simulink model "simulink_model"  (R2023a)
settings: Solver=VariableStepAuto  StartTime=0.0  StopTime=100  RelTol=1e-1
InitFcn:
  | m = 0.0489; % Mass of the drone (kg)
  | d = 0.00116; % Torque constant of one motor (N*m / s^2)
  | b = 4*1e-5; % Thrust constant of one motor (N / s^2)
  | Ixx = 48932*1e-9; % Drone inertia around the xx axis (Kg * m^2)
  | Iyy = 49929*1e-9; % Drone inertia around the yy axis (Kg * m^2)
  | Izz = 99299*1e-9; % Drone inertia around the zz axis (Kg * m^2)
  | l = 0.116 / 2; % Lenght from the motor to the mid point (m)
  | Jr = 729*1e-9; % Rotor inertia (Kg * m^2)
  | Ax = 0; % Air resistance from axis X (kg / s)
  | Ay = 0; % Air resistance from axis Y (kg / s)
  | Az = 0; % Air resistance from axis Z (kg / s)
  | g = 9.81; % The accelaration from gravity (m / s^2)
  | 
  | %Theta PID
  | Theta_P = 0;%2 * 0.6;
  | Theta_I = 0;%0.132 / 2;
  | Theta_D = 0;%0.132 / 8;
  | 
  | %Phi PID
  | Phi_P = 0;
  | Phi_I = 0;
  | Phi_D = 0;
  | 
  | %Psi_dot PID
  | Psi_dot_P = 0;
  | Psi_dot_I = 0;
  | Psi_dot_D = 0;
  | 
  | %Without noise
  | %Starting calibration Kp = 0.4
  | Z_P = 0.7 * 0.6; %0.8 * 0.6
  | Z_I = 0.99 / 2;
  | Z_D = 1.3 / 8;
libraries: slpidlib x2, sim3dlib x1, uavsim3dlib x1
settings Model: Creator=Artis  LastModifiedBy=Artis
settings OptimizationCC: ReuseModelBlockBuffer=off

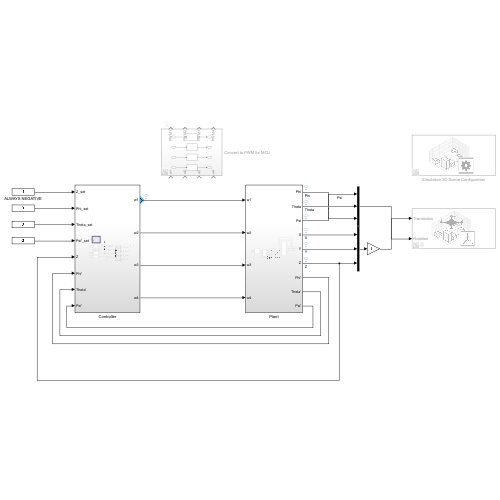
[thumbnail: Simulink's stored preview of the top-level diagram]
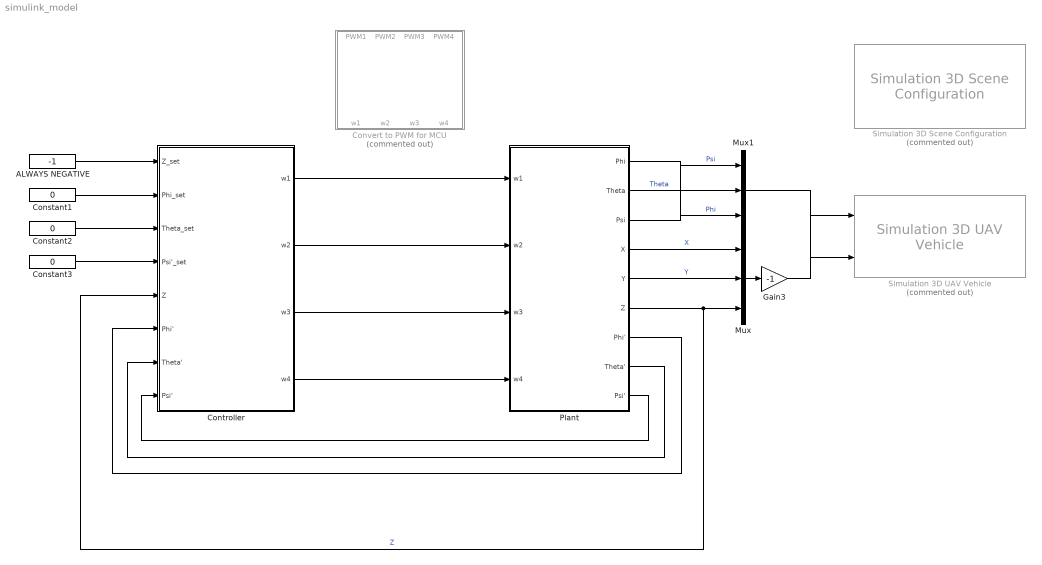
== system simulink_model ==
  ALWAYS NEGATIVE : Constant  Value=-1
  Constant1 : Constant  Value=0
  Constant2 : Constant  Value=0
  Constant3 : Constant  Value=0
  Controller : Subsystem
  Convert to PWM for MCU : Subsystem  Commented=on
  Gain3 : Gain  Gain=-1
  Mux : Mux  Inputs=3
  Mux1 : Mux  Inputs=3
  Plant : Subsystem
  Simulation 3D Scene Configuration : sim3dlib/Simulation 3D Scene Configuration  Priority=0  Commented=on  ProjectFormat=Default Scenes  SceneDesc=US city block  ProjectName=C:\Program Files\MATLAB\R2023a\toolbox\shared\sim3d_projects\automotive_project\UE4\WindowsNoEditor\VehicleSimulation.exe  ScenePath=/Game/Maps/USCityBlock  EnableOpenDRIVE=off  vehTagList={'Scene Origin';'SimulinkVehicle1'}  vehTag=SimulinkVehicle1  OpVisEn=off  Ts=1/60  EnableWindow=on  EnableRemoteAccess=off  EnableWeather=off  SunAltitude=40.0  SunAzimuth=90  clouds=10  wind=1  fog=0  rain=0  EnableGeospatial=off  OriginHeight=200  OriginLatitude=40.744652  OriginLongitude=-73.988864  MapStyle=Aerial  AdditionalAssetIDs=[]  UseAdvancedSunSky=off  SolarTime=11  TimeZone=-5  Day=21  Month=9  Year=2022  UseDaylightSavingTime=on  DSTStartDay=10  DSTStartMonth=3  DSTEndDay=3  DSTEndMonth=11  DSTSwitchHour=2  sensorTag=MainCamera1  sensorId=1  sensorName=MainCamera1  mountLoc=Origin  offsetFlag=off  tmountOffset=[0, 0, 0]  rmountOffset=[0, 0, 0]  HorizontalResolution=1280  VerticalResolution=720  HorizontalFOV=60  mountPoint=[0 0 0]  mountOrientation=[0 0 0]  aMode=4  ID=1  GeoTrigger=Inactive
      settings: LibrarySourceBlock=uavsim3dlib/Simulation 3D Scene Configuration
  Simulation 3D UAV Vehicle : uavsim3dlib/Simulation 3D UAV Vehicle  Priority=-1  Commented=on  Mesh=Quadrotor  MeshPath=/MathWorksUAVContent/UAVs/HexaRotorUAV/HexaRotor.HexaRotor  Color=Black  ActorName=SimulinkVehicle1  UseGlobalFrame=off  InitialTranslation=[0 0 0]  InitialRotation=[0 0 0]  InitialTranslationGlobal=[0 0 0]  InitialGeoOrigin=[0 0 0]  InitialRotationGlobal=[0 0 0]  SampleTime=-1  ActorType=SimulinkVehicle  ID=1  aMode=4  ActorTag=SimulinkVehicle1
  wires:
  Plant/6(Z) -> Controller/5(Z), Mux/3  "Z"
  Plant/5(Y) -> Mux/2  "Y"
  Plant/3(Psi) -> Mux1/1  "Psi"
  Plant/2(Theta) -> Mux1/2  "Theta"
  Plant/1(Phi) -> Mux1/3  "Phi"
  Plant/4(X) -> Mux/1  "X"
  Mux/1 -> Gain3/1
  Mux1/1 -> Simulation 3D UAV Vehicle/2
  Gain3/1 -> Simulation 3D UAV Vehicle/1
  ALWAYS NEGATIVE/1 -> Controller/1(Z_set)
  Constant1/1 -> Controller/2(Phi_set)
  Constant2/1 -> Controller/3(Theta_set)
  Constant3/1 -> Controller/4(Psi'_set)
  Plant/9(Psi') -> Controller/8(Psi')
  Controller/1(w1) -> Plant/1(w1)
  Controller/2(w2) -> Plant/2(w2)
  Controller/4(w4) -> Plant/4(w4)
  Controller/3(w3) -> Plant/3(w3)
  Plant/7(Phi') -> Controller/6(Phi')
  Plant/8(Theta') -> Controller/7(Theta')

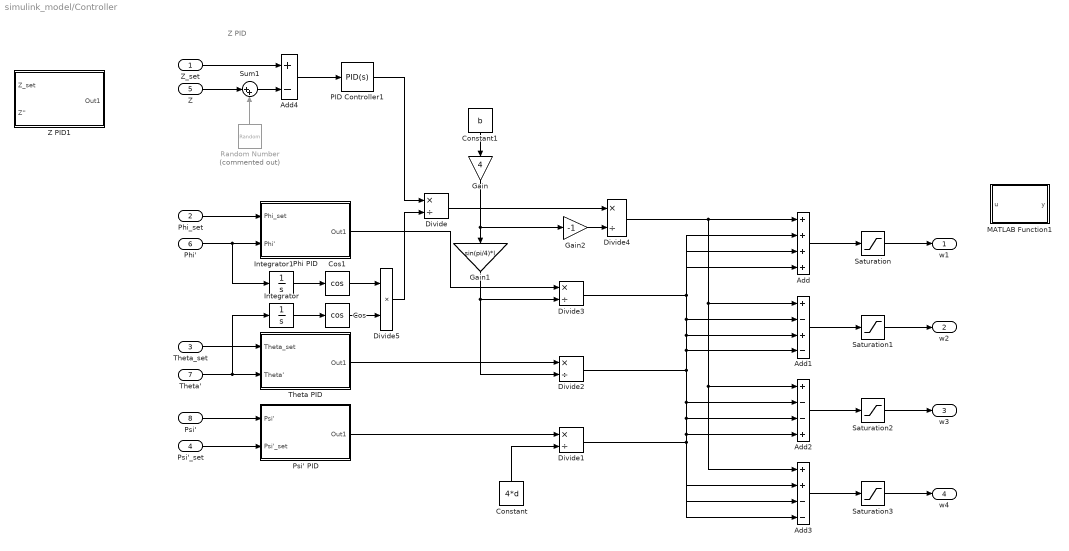
== system simulink_model/Controller ==
  note: Z PID
  Z_set : Inport
  Phi_set : Inport  Port=2
  Theta_set : Inport  Port=3
  Psi'_set : Inport  Port=4
  Z : Inport  Port=5
  Phi' : Inport  Port=6
  Theta' : Inport  Port=7
  Psi' : Inport  Port=8
  Add : Sum  Inputs=++++
  Add1 : Sum  Inputs=+-+-
  Add2 : Sum  Inputs=+--+
  Add3 : Sum  Inputs=++--
  Add4 : Sum  Inputs=+-
  Constant : Constant  Value=4*d
  Constant1 : Constant  Value=b
  Cos : Trigonometry  Operator=cos
  Cos1 : Trigonometry  Operator=cos
  Divide{,1..4} (5 alike) : Product  Inputs=*/
  Divide5 : Product  Inputs=**
  Gain : Gain  Gain=4
  Gain1 : Gain  Gain=sin(pi/4)*l
  Gain2 : Gain  Gain=-1
  Integrator : Integrator
  Integrator1 : Integrator
  MATLAB Function1 : MATLAB Function  TreatAsAtomicUnit=on
  PID Controller1 : slpidlib/PID Controller  Controller=PID  Form=Parallel  TimeDomain=Continuous-time  UseExternalTs=off  SampleTime=-1  IntegratorMethod=Forward Euler  FilterMethod=Forward Euler  ControllerParametersSource=internal  P=0.00907971597395873  I=0.000425064890164197  UseKiTs=off  D=0.0476247360001517  N=5.45397025421619  UseFilter=on  TunerSelectOption=Transfer Function Based (PID Tuner App)  InitialConditionSource=internal  InitialConditionForIntegrator=0  InitialConditionForFilter=0  DifferentiatorICPrevScaledInput=0  ExternalReset=none  TrackingMode=off  Kt=1  LimitOutput=off  SatLimitsSource=internal  UpperSaturationLimit=inf  LowerSaturationLimit=-inf  LinearizeAsGain=on  AntiWindupMode=none  Kb=1  LimitIntegrator=off  UpperIntegratorSaturationLimit=inf  LowerIntegratorSaturationLimit=-inf  POutMin=[]  POutMax=[]  IOutMin=[]  IOutMax=[]  DOutMin=[]  DOutMax=[]  NOutMin=[]  NOutMax=[]  SumOutMin=[]  SumOutMax=[]  SaturationOutMin=[]  SaturationOutMax=[]  PParamMin=[]  PParamMax=[]  IParamMin=[]  IParamMax=[]  DParamMin=[]  DParamMax=[]  NParamMin=[]  NParamMax=[]  KbParamMin=[]  KbParamMax=[]  KtParamMin=[]  KtParamMax=[]  KbOutMin=[]  KbOutMax=[]  KtOutMin=[]  KtOutMax=[]  IntegratorOutMin=[]  IntegratorOutMax=[]  FilterOutMin=[]  FilterOutMax=[]  SumI1OutMin=[]  SumI1OutMax=[]  SumI2OutMin=[]  SumI2OutMax=[]  SumI3OutMin=[]  SumI3OutMax=[]  SumI4OutMin=[]  SumI4OutMax=[]  SumDOutMin=[]  SumDOutMax=[]  DifferentiatorOutMin=[]  DifferentiatorOutMax=[]  FilterDiffOutCoefMin=[]  FilterDiffOutCoefMax=[]  ReciprocalOutMin=[]  ReciprocalOutMax=[]  SumDenOutMin=[]  SumDenOutMax=[]  SumNumOutMin=[]  SumNumOutMax=[]  DivideOutMin=[]  DivideOutMax=[]  UdiffTsProdOutMin=[]  UdiffTsProdOutMax=[]  NTsProdOutMin=[]  NTsProdOutMax=[]  UintegralTsProdOutMin=[]  UintegralTsProdOutMax=[]  UngainTsProdOutMin=[]  UngainTsProdOutMax=[]  ClampingZeroOutDataTypeStr=Inherit: Inherit via back propagation  ClampingZeroOutMin=[]  ClampingZeroOutMax=[]  FilterDenConstantOutDataTypeStr=Inherit: Inherit via back propagation  FilterDenConstantOutMin=[]  FilterDenConstantOutMax=[]  PCopyOutDataTypeStr=Inherit: Inherit via back propagation  PCopyOutMin=[]  PCopyOutMax=[]  NCopyOutDataTypeStr=Inherit: Inherit via back propagation  NCopyOutMin=[]  NCopyOutMax=[]  IntegratorContinuousStateAttributes=''  IntegratorStateMustResolveToSignalObject=off  IntegratorRTWStateStorageClass=Auto  FilterContinuousStateAttributes=''  FilterStateMustResolveToSignalObject=off  FilterRTWStateStorageClass=Auto  ParallelPVariant=InternalParameters  IdealPVariant=Disabled  IVariant=InternalParameters  DVariant=InternalParameters  IntegratorVariant=Continuous  SatVariant=Disabled  AWVariant=Passthrough  PCopyVariant=Disabled  TRVariant=Disabled  FdbkBlocksVariant=Forward  IdealPFdbkVariant=Disabled  SatFdbkVariant=Disabled  DerivativeFilterVariant=ContFilter  NVariant=InternalParameters  NCopyVariant=Disabled  FilterICVariant=InternalICsFilter  IntegratorICVariant=InternalICs  ExternalResetVariant=Disabled  TRSumVariant=Passthrough  SumFdbkVariant=Disabled  SumVariant=Sum_PID  TsampFilterVariant=InternalTs  TsampNgainVariant=Passthrough  TsampIntegralVariant=Passthrough  ExternalSaturationOutDataTypeStr=Inherit: Same as second input
  Phi PID : Subsystem
  Psi' PID : Subsystem
  Random Number : RandomNumber  Commented=on  Variance=0.001  SampleTime=0.01
  Saturation{,1..3} (4 alike) : Saturate  UpperLimit=3500  LowerLimit=0
  Sum1 : Sum  Inputs=|++
  Theta PID : Subsystem
  Z PID1 : Subsystem
  w1 : Outport
  w2 : Outport  Port=2
  w3 : Outport  Port=3
  w4 : Outport  Port=4
  wires:
  Psi'/1 -> Psi' PID/1(Psi')
  Psi'_set/1 -> Psi' PID/2(Psi'_set)
  Phi_set/1 -> Phi PID/1(Phi_set)
  Phi'/1 -> Integrator1/1, Phi PID/2(Phi')
  Theta'/1 -> Integrator/1, Theta PID/2(Theta')
  Theta_set/1 -> Theta PID/1(Theta_set)
  PID Controller1/1 -> Divide/1
  Integrator/1 -> Cos/1
  Integrator1/1 -> Cos1/1
  Divide5/1 -> Divide/2
  Cos1/1 -> Divide5/1
  Cos/1 -> Divide5/2
  Constant1/1 -> Gain/1
  Gain/1 -> Gain1/1, Gain2/1
  Gain2/1 -> Divide4/2
  Gain1/1 -> Divide3/2, Divide2/2
  Constant/1 -> Divide1/2
  Psi' PID/1(Out1) -> Divide1/1
  Divide1/1 -> Add/4, Add1/4, Add2/4, Add3/4
  Divide3/1 -> Add2/2, Add3/2, Add1/2, Add/2
  Divide2/1 -> Add2/3, Add3/3, Add/3, Add1/3
  Divide4/1 -> Add2/1, Add3/1, Add1/1, Add/1
  Theta PID/1(Out1) -> Divide2/1
  Phi PID/1(Out1) -> Divide3/1
  Divide/1 -> Divide4/1
  Add/1 -> Saturation/1
  Add1/1 -> Saturation1/1
  Add2/1 -> Saturation2/1
  Add3/1 -> Saturation3/1
  Saturation/1 -> w1/1
  Saturation1/1 -> w2/1
  Saturation2/1 -> w3/1
  Saturation3/1 -> w4/1
  Sum1/1 -> Add4/2
  Z/1 -> Sum1/1
  Random Number/1 -> Sum1/2
  Add4/1 -> PID Controller1/1
  Z_set/1 -> Add4/1

== system simulink_model/Convert to PWM for MCU ==
  w1 : Inport
  w2 : Inport  Port=2
  w3 : Inport  Port=3
  w4 : Inport  Port=4
  MATLAB Function : MATLAB Function  TreatAsAtomicUnit=on
  MATLAB Function1 : MATLAB Function  TreatAsAtomicUnit=on
  MATLAB Function2 : MATLAB Function  TreatAsAtomicUnit=on
  MATLAB Function3 : MATLAB Function  TreatAsAtomicUnit=on
  PWM1 : Outport
  PWM2 : Outport  Port=2
  PWM3 : Outport  Port=3
  PWM4 : Outport  Port=4
  wires:
  MATLAB Function1/1(y) -> PWM2/1
  w1/1 -> MATLAB Function/1(x)
  w3/1 -> MATLAB Function2/1(x)
  w2/1 -> MATLAB Function1/1(x)
  MATLAB Function2/1(y) -> PWM3/1
  MATLAB Function/1(y) -> PWM1/1
  MATLAB Function3/1(y) -> PWM4/1
  w4/1 -> MATLAB Function3/1(x)

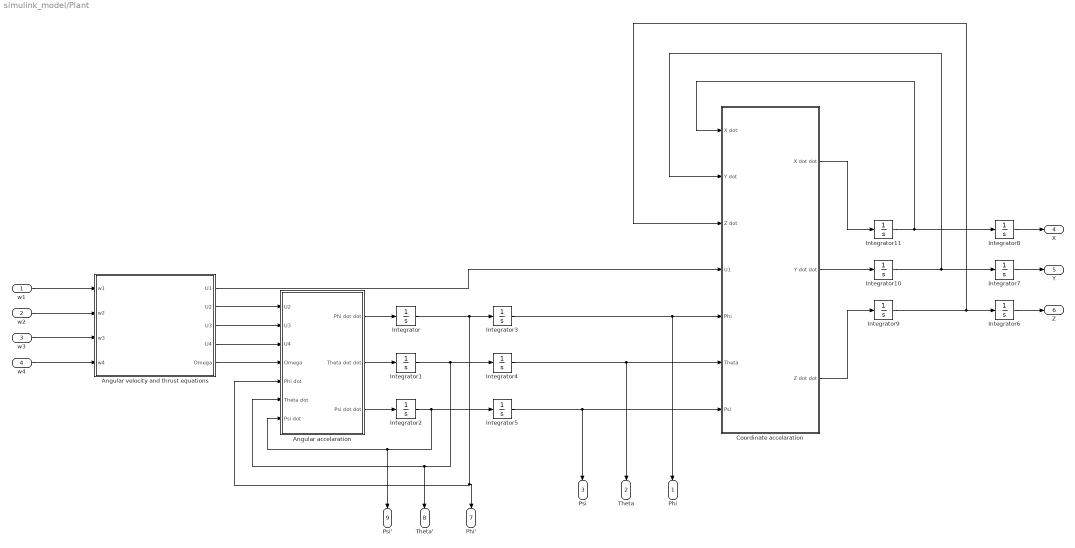
== system simulink_model/Plant ==
  w1 : Inport
  w2 : Inport  Port=2
  w3 : Inport  Port=3
  w4 : Inport  Port=4
  Angular accelaration : Subsystem
  Angular velocity and thrust equations : Subsystem
  Coordinate accelaration : Subsystem
  Integrator{,1..5,7..11} (11 alike) : Integrator
  Integrator6 : Integrator  LimitOutput=on  UpperSaturationLimit=0
  Phi : Outport
  Theta : Outport  Port=2
  Psi : Outport  Port=3
  X : Outport  Port=4
  Y : Outport  Port=5
  Z : Outport  Port=6
  Phi' : Outport  Port=7
  Theta' : Outport  Port=8
  Psi' : Outport  Port=9
  wires:
  w1/1 -> Angular velocity and thrust equations/1(w1)
  w3/1 -> Angular velocity and thrust equations/3(w3)
  Angular velocity and thrust equations/5(Omega) -> Angular accelaration/4(Omega)
  Angular velocity and thrust equations/4(U4) -> Angular accelaration/3(U4)
  Angular velocity and thrust equations/3(U3) -> Angular accelaration/2(U3)
  Angular velocity and thrust equations/2(U2) -> Angular accelaration/1(U2)
  Angular accelaration/1(Phi dot dot) -> Integrator/1
  Angular accelaration/2(Theta dot dot) -> Integrator1/1
  Angular accelaration/3(Psi dot dot) -> Integrator2/1
  Integrator/1 -> Integrator3/1, Phi'/1, Angular accelaration/5(Phi dot)
  Integrator1/1 -> Integrator4/1, Theta'/1, Angular accelaration/6(Theta dot)
  Integrator2/1 -> Integrator5/1, Psi'/1, Angular accelaration/7(Psi dot)
  Integrator4/1 -> Coordinate accelaration/6(Theta), Theta/1
  Integrator3/1 -> Coordinate accelaration/5(Phi), Phi/1
  Integrator5/1 -> Coordinate accelaration/7(Psi), Psi/1
  Angular velocity and thrust equations/1(U1) -> Coordinate accelaration/4(U1)
  Integrator6/1 -> Z/1
  Integrator7/1 -> Y/1
  Integrator8/1 -> X/1
  Integrator10/1 -> Integrator7/1, Coordinate accelaration/2(Y dot)
  Integrator9/1 -> Integrator6/1, Coordinate accelaration/3(Z dot)
  Integrator11/1 -> Integrator8/1, Coordinate accelaration/1(X dot)
  Coordinate accelaration/1(X dot dot) -> Integrator11/1
  Coordinate accelaration/2(Y dot dot) -> Integrator10/1
  Coordinate accelaration/3(Z dot dot) -> Integrator9/1
  w2/1 -> Angular velocity and thrust equations/2(w2)
  w4/1 -> Angular velocity and thrust equations/4(w4)

== system simulink_model/Controller/Phi PID ==
  Phi_set : Inport
  Phi' : Inport  Port=2
  Add : Sum  Inputs=+-
  Add1 : Sum  Inputs=++-
  Gain : Gain  Gain=Phi_P
  Gain1 : Gain  Gain=Phi_I
  Gain2 : Gain  Gain=Phi_D
  Integrator : Integrator
  Integrator1 : Integrator
  Out1 : Outport
  wires:
  Phi_set/1 -> Add/1
  Add1/1 -> Out1/1
  Gain/1 -> Add1/1
  Add/1 -> Gain/1, Integrator/1
  Integrator/1 -> Gain1/1
  Gain1/1 -> Add1/2
  Gain2/1 -> Add1/3
  Phi'/1 -> Gain2/1, Integrator1/1
  Integrator1/1 -> Add/2

== system simulink_model/Controller/Psi' PID ==
  Psi' : Inport
  Psi'_set : Inport  Port=2
  Add : Sum  Inputs=-+
  Add1 : Sum  Inputs=+++
  Derivative : Derivative
  Gain : Gain  Gain=Psi_dot_P
  Gain1 : Gain  Gain=Psi_dot_I
  Gain2 : Gain  Gain=Psi_dot_D
  Integrator : Integrator
  Out1 : Outport
  wires:
  Psi'/1 -> Add/1
  Psi'_set/1 -> Add/2
  Add1/1 -> Out1/1
  Gain/1 -> Add1/1
  Integrator/1 -> Gain1/1
  Gain1/1 -> Add1/2
  Gain2/1 -> Add1/3
  Add/1 -> Derivative/1, Gain/1, Integrator/1
  Derivative/1 -> Gain2/1

== system simulink_model/Controller/Theta PID ==
  Theta_set : Inport
  Theta' : Inport  Port=2
  Add : Sum  Inputs=+-
  Add1 : Sum  Inputs=++-
  Gain : Gain  Gain=Theta_P
  Gain1 : Gain  Gain=Theta_I
  Gain2 : Gain  Gain=Theta_D
  Integrator : Integrator
  Integrator1 : Integrator
  Random Number : RandomNumber  SampleTime=0.1
  Sum : Sum  Inputs=|++
  Out1 : Outport
  wires:
  Theta_set/1 -> Add/1
  Add1/1 -> Out1/1
  Gain/1 -> Add1/1
  Add/1 -> Sum/1, Integrator/1
  Integrator/1 -> Gain1/1
  Gain1/1 -> Add1/2
  Gain2/1 -> Add1/3
  Theta'/1 -> Gain2/1, Integrator1/1
  Integrator1/1 -> Add/2
  Sum/1 -> Gain/1
  Random Number/1 -> Sum/2

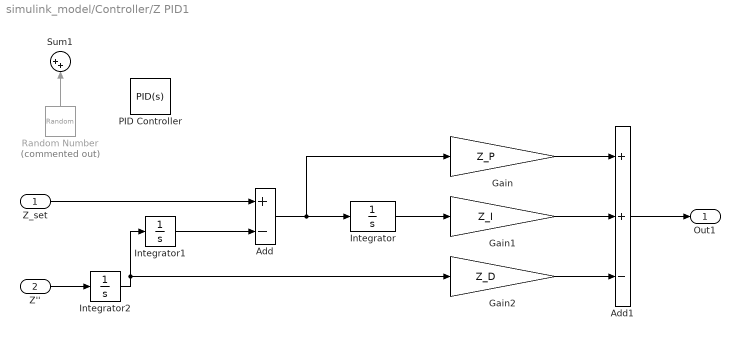
== system simulink_model/Controller/Z PID1 ==
  Z_set : Inport
  Z'' : Inport  Port=2
  Add : Sum  Inputs=+-
  Add1 : Sum  Inputs=++-
  Gain : Gain  Gain=Z_P
  Gain1 : Gain  Gain=Z_I
  Gain2 : Gain  Gain=Z_D
  Integrator : Integrator
  Integrator1 : Integrator  LimitOutput=on  UpperSaturationLimit=0
  Integrator2 : Integrator
  PID Controller : slpidlib/PID Controller  Controller=PID  Form=Parallel  TimeDomain=Continuous-time  UseExternalTs=off  SampleTime=-1  IntegratorMethod=Forward Euler  FilterMethod=Forward Euler  ControllerParametersSource=internal  P=1  I=1  UseKiTs=off  D=0  N=100  UseFilter=on  TunerSelectOption=Transfer Function Based (PID Tuner App)  InitialConditionSource=internal  InitialConditionForIntegrator=0  InitialConditionForFilter=0  DifferentiatorICPrevScaledInput=0  ExternalReset=none  TrackingMode=off  Kt=1  LimitOutput=off  SatLimitsSource=internal  UpperSaturationLimit=inf  LowerSaturationLimit=-inf  LinearizeAsGain=on  AntiWindupMode=none  Kb=1  LimitIntegrator=off  UpperIntegratorSaturationLimit=inf  LowerIntegratorSaturationLimit=-inf  POutMin=[]  POutMax=[]  IOutMin=[]  IOutMax=[]  DOutMin=[]  DOutMax=[]  NOutMin=[]  NOutMax=[]  SumOutMin=[]  SumOutMax=[]  SaturationOutMin=[]  SaturationOutMax=[]  PParamMin=[]  PParamMax=[]  IParamMin=[]  IParamMax=[]  DParamMin=[]  DParamMax=[]  NParamMin=[]  NParamMax=[]  KbParamMin=[]  KbParamMax=[]  KtParamMin=[]  KtParamMax=[]  KbOutMin=[]  KbOutMax=[]  KtOutMin=[]  KtOutMax=[]  IntegratorOutMin=[]  IntegratorOutMax=[]  FilterOutMin=[]  FilterOutMax=[]  SumI1OutMin=[]  SumI1OutMax=[]  SumI2OutMin=[]  SumI2OutMax=[]  SumI3OutMin=[]  SumI3OutMax=[]  SumI4OutMin=[]  SumI4OutMax=[]  SumDOutMin=[]  SumDOutMax=[]  DifferentiatorOutMin=[]  DifferentiatorOutMax=[]  FilterDiffOutCoefMin=[]  FilterDiffOutCoefMax=[]  ReciprocalOutMin=[]  ReciprocalOutMax=[]  SumDenOutMin=[]  SumDenOutMax=[]  SumNumOutMin=[]  SumNumOutMax=[]  DivideOutMin=[]  DivideOutMax=[]  UdiffTsProdOutMin=[]  UdiffTsProdOutMax=[]  NTsProdOutMin=[]  NTsProdOutMax=[]  UintegralTsProdOutMin=[]  UintegralTsProdOutMax=[]  UngainTsProdOutMin=[]  UngainTsProdOutMax=[]  ClampingZeroOutDataTypeStr=Inherit: Inherit via back propagation  ClampingZeroOutMin=[]  ClampingZeroOutMax=[]  FilterDenConstantOutDataTypeStr=Inherit: Inherit via back propagation  FilterDenConstantOutMin=[]  FilterDenConstantOutMax=[]  PCopyOutDataTypeStr=Inherit: Inherit via back propagation  PCopyOutMin=[]  PCopyOutMax=[]  NCopyOutDataTypeStr=Inherit: Inherit via back propagation  NCopyOutMin=[]  NCopyOutMax=[]  IntegratorContinuousStateAttributes=''  IntegratorStateMustResolveToSignalObject=off  IntegratorRTWStateStorageClass=Auto  FilterContinuousStateAttributes=''  FilterStateMustResolveToSignalObject=off  FilterRTWStateStorageClass=Auto  ParallelPVariant=InternalParameters  IdealPVariant=Disabled  IVariant=InternalParameters  DVariant=InternalParameters  IntegratorVariant=Continuous  SatVariant=Disabled  AWVariant=Passthrough  PCopyVariant=Disabled  TRVariant=Disabled  FdbkBlocksVariant=Forward  IdealPFdbkVariant=Disabled  SatFdbkVariant=Disabled  DerivativeFilterVariant=ContFilter  NVariant=InternalParameters  NCopyVariant=Disabled  FilterICVariant=InternalICsFilter  IntegratorICVariant=InternalICs  ExternalResetVariant=Disabled  TRSumVariant=Passthrough  SumFdbkVariant=Disabled  SumVariant=Sum_PID  TsampFilterVariant=InternalTs  TsampNgainVariant=Passthrough  TsampIntegralVariant=Passthrough  ExternalSaturationOutDataTypeStr=Inherit: Same as second input
  Random Number : RandomNumber  Commented=on  Variance=0.001  SampleTime=0.01
  Sum1 : Sum  Inputs=|++
  Out1 : Outport
  wires:
  Z_set/1 -> Add/1
  Add1/1 -> Out1/1
  Gain/1 -> Add1/1
  Integrator/1 -> Gain1/1
  Gain1/1 -> Add1/2
  Gain2/1 -> Add1/3
  Z''/1 -> Integrator2/1
  Add/1 -> Gain/1, Integrator/1
  Integrator2/1 -> Gain2/1, Integrator1/1
  Random Number/1 -> Sum1/2
  Integrator1/1 -> Add/2

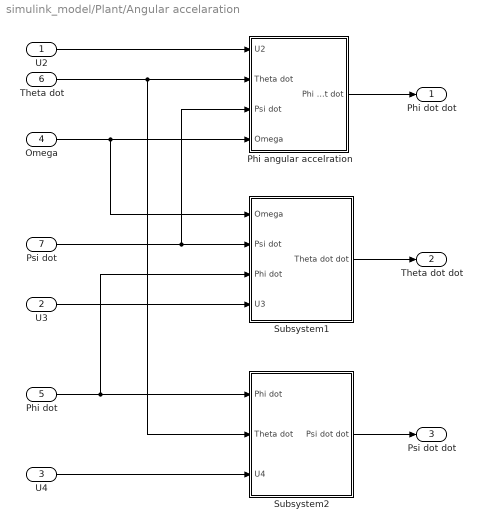
== system simulink_model/Plant/Angular accelaration ==
  U2 : Inport
  U3 : Inport  Port=2
  U4 : Inport  Port=3
  Omega : Inport  Port=4
  Phi dot : Inport  Port=5
  Theta dot : Inport  Port=6
  Psi dot : Inport  Port=7
  Phi angular accelration : Subsystem
  Subsystem1 : Subsystem
  Subsystem2 : Subsystem
  Phi dot dot : Outport
  Theta dot dot : Outport  Port=2
  Psi dot dot : Outport  Port=3
  wires:
  Phi angular accelration/1(Phi dot dot) -> Phi dot dot/1
  Subsystem1/1(Theta dot dot) -> Theta dot dot/1
  Subsystem2/1(Psi dot dot) -> Psi dot dot/1
  U2/1 -> Phi angular accelration/1(U2)
  Theta dot/1 -> Subsystem2/2(Theta dot), Phi angular accelration/2(Theta dot)
  Psi dot/1 -> Phi angular accelration/3(Psi dot), Subsystem1/2(Psi dot)
  Omega/1 -> Subsystem1/1(Omega), Phi angular accelration/4(Omega)
  U3/1 -> Subsystem1/4(U3)
  Phi dot/1 -> Subsystem1/3(Phi dot), Subsystem2/1(Phi dot)
  U4/1 -> Subsystem2/3(U4)

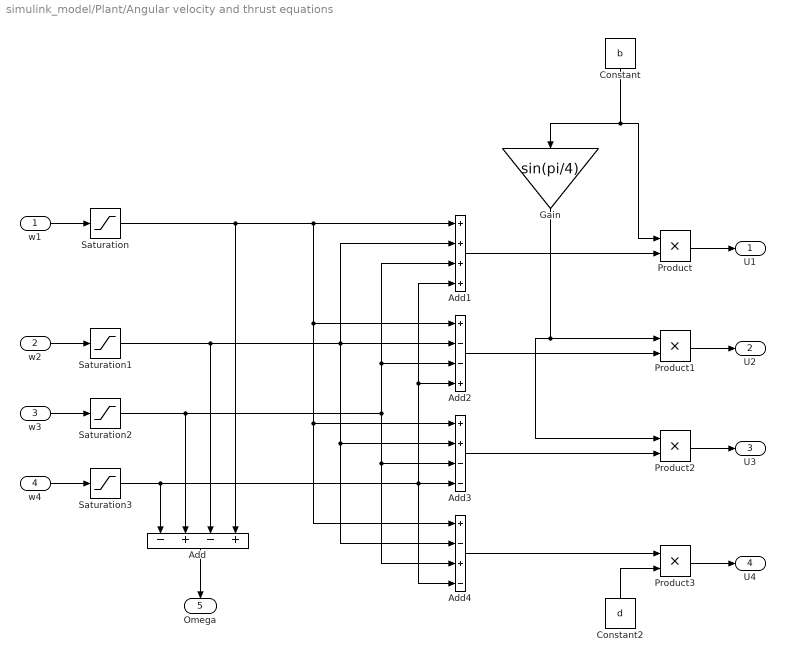
== system simulink_model/Plant/Angular velocity and thrust equations ==
  w1 : Inport
  w2 : Inport  Port=2
  w3 : Inport  Port=3
  w4 : Inport  Port=4
  Add : Sum  Inputs=-+-+
  Add1 : Sum  Inputs=++++
  Add2 : Sum  Inputs=+--+
  Add3 : Sum  Inputs=++--
  Add4 : Sum  Inputs=+-+-
  Constant : Constant  Value=b
  Constant2 : Constant  Value=d
  Gain : Gain  Gain=sin(pi/4)
  Product{,1..3} (4 alike) : Product
  Saturation{,1..3} (4 alike) : Saturate  UpperLimit=inf  LowerLimit=0
  U1 : Outport
  U2 : Outport  Port=2
  U3 : Outport  Port=3
  U4 : Outport  Port=4
  Omega : Outport  Port=5
  wires:
  Add/1 -> Omega/1
  w1/1 -> Saturation/1
  w2/1 -> Saturation1/1
  w3/1 -> Saturation2/1
  w4/1 -> Saturation3/1
  Product/1 -> U1/1
  Add1/1 -> Product/2
  Add4/1 -> Product3/1
  Add3/1 -> Product2/2
  Add2/1 -> Product1/2
  Constant2/1 -> Product3/2
  Gain/1 -> Product2/1, Product1/1
  Product3/1 -> U4/1
  Product2/1 -> U3/1
  Product1/1 -> U2/1
  Constant/1 -> Product/1, Gain/1
  Saturation/1 -> Add1/1, Add2/1, Add3/1, Add4/1, Add/4
  Saturation1/1 -> Add3/2, Add4/2, Add2/2, Add1/2, Add/3
  Saturation2/1 -> Add/2, Add1/3, Add2/3, Add3/3, Add4/3
  Saturation3/1 -> Add4/4, Add2/4, Add1/4, Add3/4, Add/1

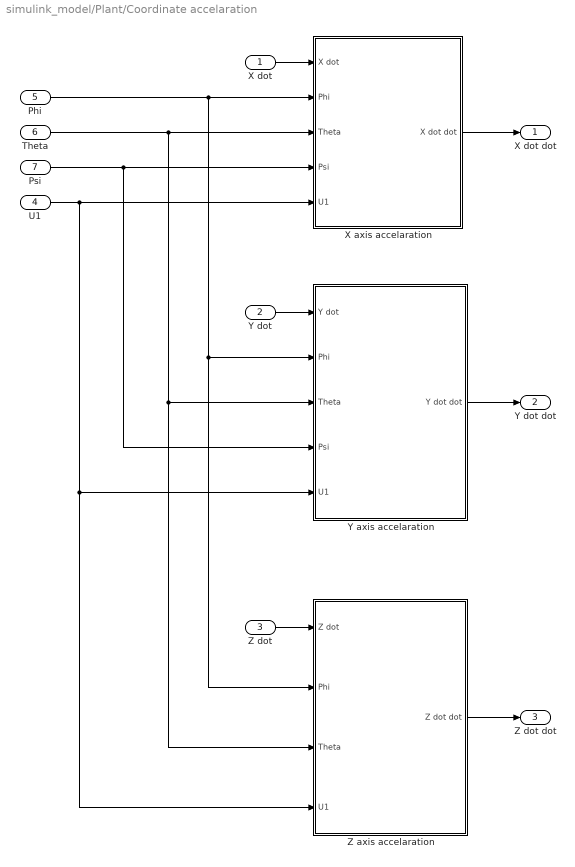
== system simulink_model/Plant/Coordinate accelaration ==
  X dot : Inport
  Y dot : Inport  Port=2
  Z dot : Inport  Port=3
  U1 : Inport  Port=4
  Phi : Inport  Port=5
  Theta : Inport  Port=6
  Psi : Inport  Port=7
  X axis accelaration : Subsystem
  Y axis accelaration : Subsystem
  Z axis accelaration : Subsystem
  X dot dot : Outport
  Y dot dot : Outport  Port=2
  Z dot dot : Outport  Port=3
  wires:
  X dot/1 -> X axis accelaration/1(X dot)
  Phi/1 -> Z axis accelaration/2(Phi), Y axis accelaration/2(Phi), X axis accelaration/2(Phi)
  Theta/1 -> Z axis accelaration/3(Theta), Y axis accelaration/3(Theta), X axis accelaration/3(Theta)
  Psi/1 -> Y axis accelaration/4(Psi), X axis accelaration/4(Psi)
  X axis accelaration/1(X dot dot) -> X dot dot/1
  U1/1 -> Z axis accelaration/4(U1), Y axis accelaration/5(U1), X axis accelaration/5(U1)
  Z axis accelaration/1(Z dot dot) -> Z dot dot/1
  Y axis accelaration/1(Y dot dot) -> Y dot dot/1
  Y dot/1 -> Y axis accelaration/1(Y dot)
  Z dot/1 -> Z axis accelaration/1(Z dot)

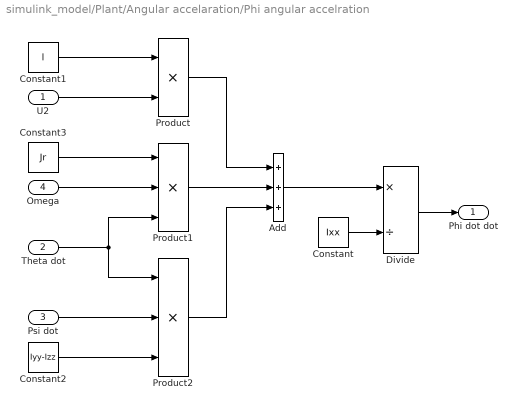
== system simulink_model/Plant/Angular accelaration/Phi angular accelration ==
  U2 : Inport
  Theta dot : Inport  Port=2
  Psi dot : Inport  Port=3
  Omega : Inport  Port=4
  Add : Sum  Inputs=+++
  Constant : Constant  Value=Ixx
  Constant1 : Constant  Value=l
  Constant2 : Constant  Value=Iyy-Izz
  Constant3 : Constant  Value=Jr
  Divide : Product  Inputs=*/
  Product : Product
  Product1 : Product  Inputs=3
  Product2 : Product  Inputs=3
  Phi dot dot : Outport
  wires:
  Divide/1 -> Phi dot dot/1
  Constant/1 -> Divide/2
  U2/1 -> Product/2
  Constant1/1 -> Product/1
  Product/1 -> Add/1
  Product1/1 -> Add/2
  Omega/1 -> Product1/2
  Theta dot/1 -> Product2/1, Product1/3
  Psi dot/1 -> Product2/2
  Constant2/1 -> Product2/3
  Product2/1 -> Add/3
  Constant3/1 -> Product1/1
  Add/1 -> Divide/1

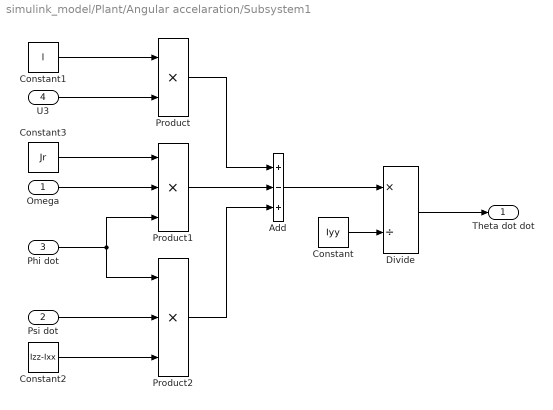
== system simulink_model/Plant/Angular accelaration/Subsystem1 ==
  Omega : Inport
  Psi dot : Inport  Port=2
  Phi dot : Inport  Port=3
  U3 : Inport  Port=4
  Add : Sum  Inputs=+-+
  Constant : Constant  Value=Iyy
  Constant1 : Constant  Value=l
  Constant2 : Constant  Value=Izz-Ixx
  Constant3 : Constant  Value=Jr
  Divide : Product  Inputs=*/
  Product : Product
  Product1 : Product  Inputs=3
  Product2 : Product  Inputs=3
  Theta dot dot : Outport
  wires:
  Constant3/1 -> Product1/1
  Psi dot/1 -> Product2/2
  Product/1 -> Add/1
  U3/1 -> Product/2
  Add/1 -> Divide/1
  Omega/1 -> Product1/2
  Phi dot/1 -> Product1/3, Product2/1
  Product1/1 -> Add/2
  Product2/1 -> Add/3
  Constant/1 -> Divide/2
  Constant1/1 -> Product/1
  Constant2/1 -> Product2/3
  Divide/1 -> Theta dot dot/1

== system simulink_model/Plant/Angular accelaration/Subsystem2 ==
  Phi dot : Inport
  Theta dot : Inport  Port=2
  U4 : Inport  Port=3
  Add : Sum
  Constant : Constant  Value=Izz
  Constant2 : Constant  Value=Ixx-Iyy
  Divide : Product  Inputs=*/
  Product1 : Product  Inputs=3
  Psi dot dot : Outport
  wires:
  Theta dot/1 -> Product1/1
  Phi dot/1 -> Product1/2
  Add/1 -> Divide/1
  Product1/1 -> Add/2
  Constant/1 -> Divide/2
  Divide/1 -> Psi dot dot/1
  U4/1 -> Add/1
  Constant2/1 -> Product1/3

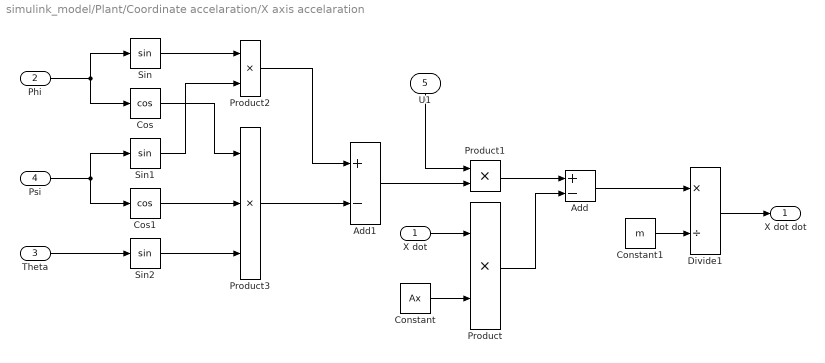
== system simulink_model/Plant/Coordinate accelaration/X axis accelaration ==
  X dot : Inport
  Phi : Inport  Port=2
  Theta : Inport  Port=3
  Psi : Inport  Port=4
  U1 : Inport  Port=5
  Add : Sum  Inputs=+-
  Add1 : Sum  Inputs=+-
  Constant : Constant  Value=Ax
  Constant1 : Constant  Value=m
  Cos : Trigonometry  Operator=cos
  Cos1 : Trigonometry  Operator=cos
  Divide1 : Product  Inputs=*/
  Product : Product
  Product1 : Product
  Product2 : Product
  Product3 : Product  Inputs=3
  Sin : Trigonometry
  Sin1 : Trigonometry
  Sin2 : Trigonometry
  X dot dot : Outport
  wires:
  Phi/1 -> Sin/1, Cos/1
  Psi/1 -> Cos1/1, Sin1/1
  Theta/1 -> Sin2/1
  X dot/1 -> Product/1
  Constant1/1 -> Divide1/2
  Constant/1 -> Product/2
  Product/1 -> Add/2
  Product1/1 -> Add/1
  U1/1 -> Product1/1
  Add1/1 -> Product1/2
  Sin/1 -> Product2/1
  Sin1/1 -> Product2/2
  Cos/1 -> Product3/1
  Cos1/1 -> Product3/2
  Sin2/1 -> Product3/3
  Product3/1 -> Add1/2
  Product2/1 -> Add1/1
  Divide1/1 -> X dot dot/1
  Add/1 -> Divide1/1

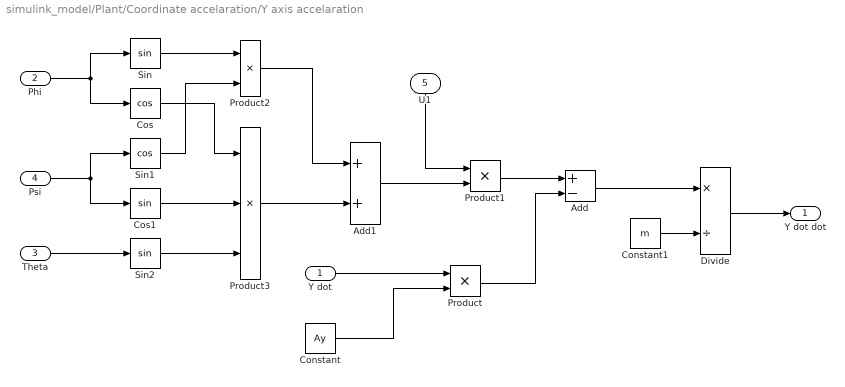
== system simulink_model/Plant/Coordinate accelaration/Y axis accelaration ==
  Y dot : Inport
  Phi : Inport  Port=2
  Theta : Inport  Port=3
  Psi : Inport  Port=4
  U1 : Inport  Port=5
  Add : Sum  Inputs=+-
  Add1 : Sum
  Constant : Constant  Value=Ay
  Constant1 : Constant  Value=m
  Cos : Trigonometry  Operator=cos
  Cos1 : Trigonometry
  Divide : Product  Inputs=*/
  Product : Product
  Product1 : Product
  Product2 : Product
  Product3 : Product  Inputs=3
  Sin : Trigonometry
  Sin1 : Trigonometry  Operator=cos
  Sin2 : Trigonometry
  Y dot dot : Outport
  wires:
  Theta/1 -> Sin2/1
  Sin/1 -> Product2/1
  Product1/1 -> Add/1
  Cos1/1 -> Product3/2
  Cos/1 -> Product3/1
  Sin1/1 -> Product2/2
  Psi/1 -> Cos1/1, Sin1/1
  Sin2/1 -> Product3/3
  Add1/1 -> Product1/2
  Y dot/1 -> Product/1
  Product2/1 -> Add1/1
  U1/1 -> Product1/1
  Product3/1 -> Add1/2
  Product/1 -> Add/2
  Phi/1 -> Sin/1, Cos/1
  Constant/1 -> Product/2
  Divide/1 -> Y dot dot/1
  Constant1/1 -> Divide/2
  Add/1 -> Divide/1

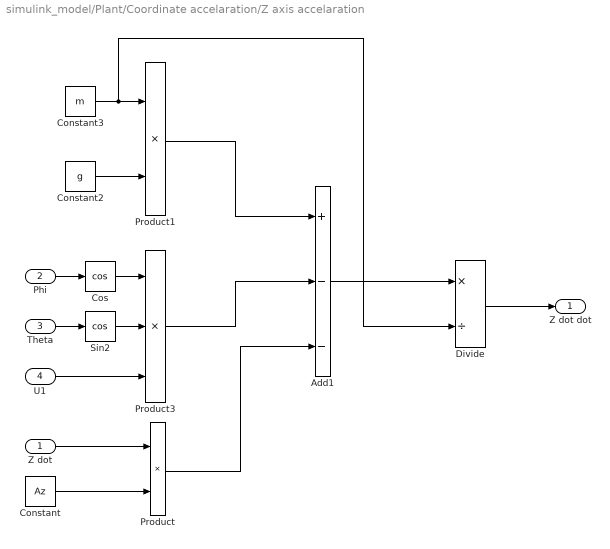
== system simulink_model/Plant/Coordinate accelaration/Z axis accelaration ==
  Z dot : Inport
  Phi : Inport  Port=2
  Theta : Inport  Port=3
  U1 : Inport  Port=4
  Add1 : Sum  Inputs=+--
  Constant : Constant  Value=Az
  Constant2 : Constant  Value=g
  Constant3 : Constant  Value=m
  Cos : Trigonometry  Operator=cos
  Divide : Product  Inputs=*/
  Product : Product
  Product1 : Product
  Product3 : Product  Inputs=3
  Sin2 : Trigonometry  Operator=cos
  Z dot dot : Outport
  wires:
  Theta/1 -> Sin2/1
  Cos/1 -> Product3/1
  Constant/1 -> Product/2
  Sin2/1 -> Product3/2
  Z dot/1 -> Product/1
  Product3/1 -> Add1/2
  Product/1 -> Add1/3
  Phi/1 -> Cos/1
  U1/1 -> Product3/3
  Divide/1 -> Z dot dot/1
  Constant3/1 -> Divide/2, Product1/1
  Add1/1 -> Divide/1
  Constant2/1 -> Product1/2
  Product1/1 -> Add1/1

== matlab function simulink_model/Convert to PWM for MCU/MATLAB Function2 ==
  data: x input; y output
function y = fcn(x)

y =  8.679e-15*x^9 -9.4e-12*x^8 + 4.063e-09*x^7 -8.819e-07*x^6 + 9.718e-05*x^5 -0.004292*x^4 -0.07222*x^3 + 10.47*x^2 + 30.47*x -1161;

== matlab function simulink_model/Convert to PWM for MCU/MATLAB Function3 ==
  data: x input; y output
function y = fcn(x)

y =  8.679e-15*x^9 -9.4e-12*x^8 + 4.063e-09*x^7 -8.819e-07*x^6 + 9.718e-05*x^5 -0.004292*x^4 -0.07222*x^3 + 10.47*x^2 + 30.47*x -1161;

== matlab function simulink_model/Controller/MATLAB Function1 ==
  data: u input; y output
function y = fcn(u)
    if 0.0795*u - 21.961 > 255
        q = 255;
    elseif 0.0795*u - 21.961 < 0
        q = 0;
    else
        q = (0.0795*u - 21.961);
    end
y = q;

== matlab function simulink_model/Convert to PWM for MCU/MATLAB Function ==
  data: x input; y output
function y = fcn(x)

y =  8.679e-15*x^9 -9.4e-12*x^8 + 4.063e-09*x^7 -8.819e-07*x^6 + 9.718e-05*x^5 -0.004292*x^4 -0.07222*x^3 + 10.47*x^2 + 30.47*x -1161;

== matlab function simulink_model/Convert to PWM for MCU/MATLAB Function1 ==
  data: x input; y output
function y = fcn(x)

y =  8.679e-15*x^9 -9.4e-12*x^8 + 4.063e-09*x^7 -8.819e-07*x^6 + 9.718e-05*x^5 -0.004292*x^4 -0.07222*x^3 + 10.47*x^2 + 30.47*x -1161;
